simulink model "StateFlow_3"  (R2018a)
settings: Solver=FixedStepDiscrete  StartTime=0.0  StopTime=10.0  FixedStep=0.01  RelTol=1e-3
settings Model: SnapshotBufferSize=1000  Creator=Choaib ELMADI  LastModifiedBy=Choaib ELMADI

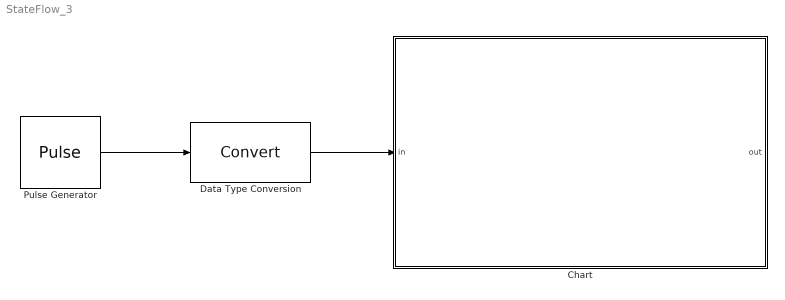
== system StateFlow_3 ==
  Chart : Stateflow chart  TreatAsAtomicUnit=on
  Data Type Conversion : DataTypeConversion
  Pulse Generator : DiscretePulseGenerator  PulseType=Time based  Period=0.1  PulseWidth=50
  wires:
  Pulse Generator/1 -> Data Type Conversion/1
  Data Type Conversion/1 -> Chart/1(in)

== stateflow chart StateFlow_3/Chart ==
  (default) -> (junction 3)
  (junction 3) -> (junction 5) [order 1] : [in==1]
  (junction 3) -> (junction 9) [order 2] : {out=0;}
  (junction 5) -> (junction 7) : {out=in+1;}
  (junction 7) -> (junction 9)
  (junction 9) -> (junction 17)
  data: in input double; out output double
